simulink subsystem "PieroControladoZ"  (R2023b)
settings: Solver=VariableStepAuto  StartTime=0.0  StopTime=10.0  RelTol=1e-3
settings Model: Creator=USUARIO  LastModifiedBy=USUARIO

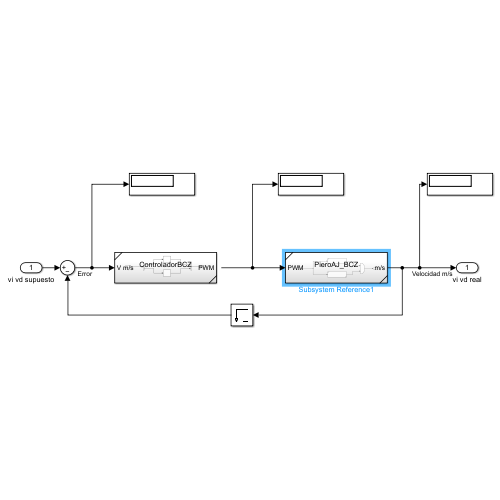
[thumbnail: Simulink's stored preview of the top-level diagram]
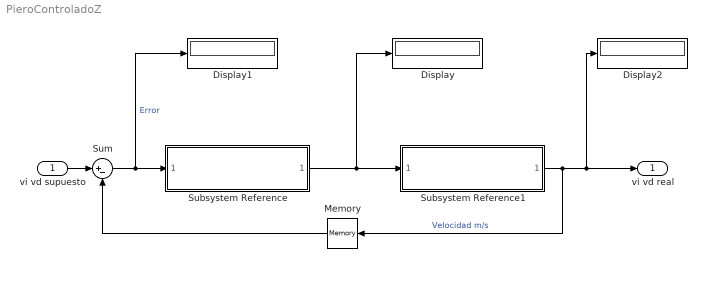
== system PieroControladoZ ==
  vi vd supuesto : Inport
  Display : Display
  Display1 : Display
  Display2 : Display
  Memory : Memory
  Subsystem Reference : Subsystem  ReferencedSubsystem=ControladorBCZ
  Subsystem Reference1 : Subsystem  ReferencedSubsystem=PieroAJ_BCZ
  Sum : Sum  Inputs=|+-
  vi vd real : Outport
  wires:
  Sum/1 -> Display1/1, Subsystem Reference/1  "Error"
  vi vd supuesto/1 -> Sum/1
  Subsystem Reference/1 -> Display/1, Subsystem Reference1/1
  Subsystem Reference1/1 -> vi vd real/1, Display2/1, Memory/1  "Velocidad m/s"
  Memory/1 -> Sum/2
